simulink model "twotankssim"  (Simulink 5.1)
settings: Solver=ode45  StartTime=0.0  StopTime=1000  RelTol=1e-3
libraries: mpt_sim x4
settings Model: LastModifiedBy=michal  BooleanDataType=on

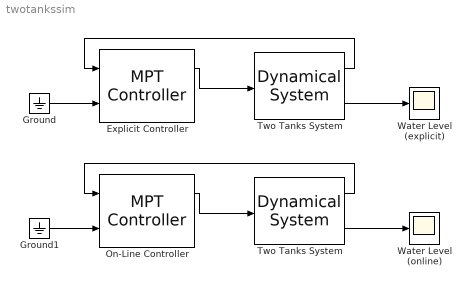
== system twotankssim ==
  Explicit Controller : mpt_sim/MPT Controller  ctrl=expc  Ts=[]  infbreak=on
  Ground : Ground
  Ground1 : Ground
  On-Line Controller : mpt_sim/MPT Controller  ctrl=onlc  Ts=[]  infbreak=on
  Two Tanks System : mpt_sim/Dynamical System  sysStruct=sysStruct  x0=[0; 0]  Ts=[]  constr=on
  "Two Tanks System " : mpt_sim/Dynamical System  sysStruct=sysStruct  x0=[0; 0]  Ts=[]  constr=on
  Water Level (explicit) : Scope
      settings: TimeRange=1000  YMin=0  YMax=0.25  SaveToWorkspace=off  SaveName=ScopeData  LimitDataPoints=on  MaxDataPoints=5000
  Water Level (online) : Scope
      settings: TimeRange=1000  YMin=0  YMax=0.25  SaveToWorkspace=off  LimitDataPoints=on  MaxDataPoints=5000
  wires:
  Ground/1 -> Explicit Controller/2
  Two Tanks System/1 -> Explicit Controller/1
  Two Tanks System/2 -> Water Level (explicit)/1
  Explicit Controller/1 -> Two Tanks System/1
  Ground1/1 -> On-Line Controller/2
  "Two Tanks System "/1 -> On-Line Controller/1
  "Two Tanks System "/2 -> Water Level (online)/1
  On-Line Controller/1 -> "Two Tanks System "/1
